simulink subsystem "Gyro_Angles"  (R2023b)
settings: Solver=VariableStepAuto  StartTime=0.0  StopTime=10.0  RelTol=1e-3
undefined symbols (not defined in the file): Gyro_Calibration_Reset_Degree, Gyro_Calibration_Reset_Flag
libraries: simulink_extras x1, simulink x1
settings Model: Creator=ander  LastModifiedBy=ander

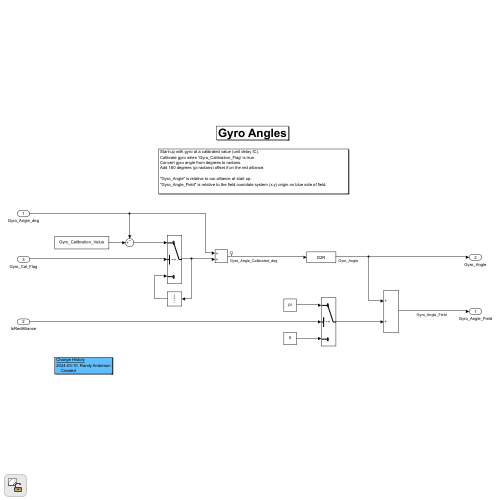
[thumbnail: Simulink's stored preview of the top-level diagram]
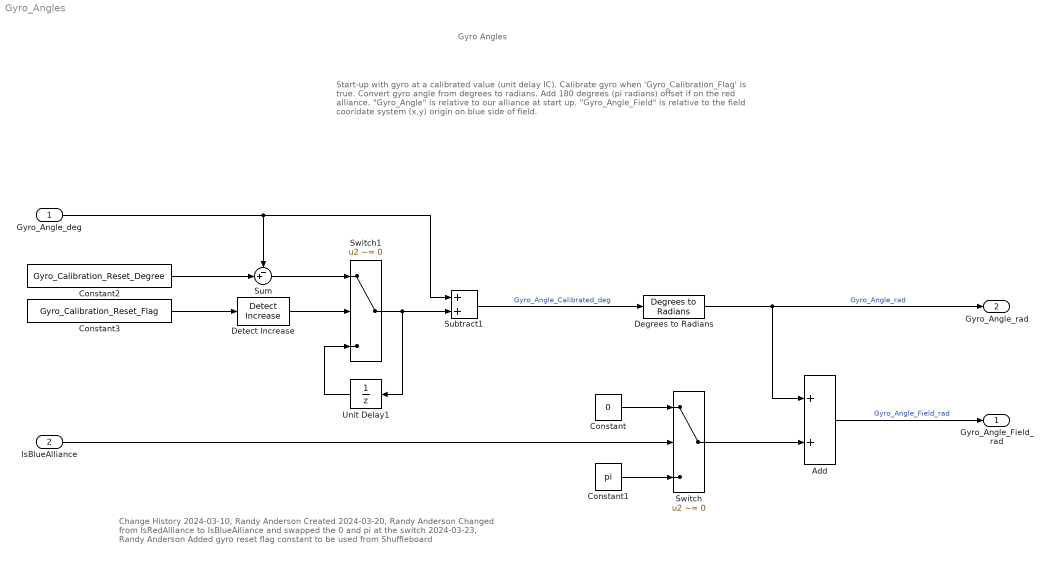
== system Gyro_Angles ==
  note: Gyro Angles
  note: Start-up with gyro at a calibrated value (unit delay IC).
      | Calibrate gyro when 'Gyro_Calibration_Flag' is true.
      | Convert gyro angle from degrees to radians.
      | Add 180 degrees (pi radians) offset if on the red alliance.
      |
      | "Gyro_Angle" is relative to our alliance at start up.
      | "Gyro_Angle_Field" is relative to the field cooridate system (x,y) origin on blue side of field.
  note: Change History
      | 2024-03-10, Randy Anderson
      | Created
      | 2024-03-20, Randy Anderson
      | Changed from IsRedAlliance to IsBlueAlliance and swapped the 0 and pi at the switch
      | 2024-03-23, Randy Anderson
      | Added gyro reset flag constant to be used from Shuffleboard
  Gyro_Angle_deg : Inport
  IsBlueAlliance : Inport  Port=2
  Add : Sum
  Constant : Constant  Value=0
  Constant1 : Constant  Value=pi
  Constant2 : Constant  Value=Gyro_Calibration_Reset_Degree
  Constant3 : Constant  Value=Gyro_Calibration_Reset_Flag
  Degrees to Radians : simulink_extras/Transformations/Degrees to Radians
  Detect Increase : simulink/Logic and Bit Operations/Detect Increase  vinit=0.0  OutDataTypeStr=boolean
  Subtract1 : Sum
  Sum : Sum  Inputs=-+|
  Switch : Switch  Criteria=u2 ~= 0  SaturateOnIntegerOverflow=off  InputSameDT=off
  Switch1 : Switch  Criteria=u2 ~= 0  SaturateOnIntegerOverflow=off  InputSameDT=off
  Unit Delay1 : UnitDelay  InitialCondition=Gyro_Calibration_Reset_Degree  SampleTime=-1  HasFrameUpgradeWarning=on
  Gyro_Angle_Field_rad : Outport
  Gyro_Angle_rad : Outport  Port=2
  wires:
  Add/1 -> Gyro_Angle_Field_rad/1  "Gyro_Angle_Field_rad"
  Degrees to Radians/1 -> Gyro_Angle_rad/1, Add/1  "Gyro_Angle_rad"
  IsBlueAlliance/1 -> Switch/2
  Constant/1 -> Switch/1
  Constant1/1 -> Switch/3
  Unit Delay1/1 -> Switch1/3
  Switch1/1 -> Subtract1/2, Unit Delay1/1
  Sum/1 -> Switch1/1
  Subtract1/1 -> Degrees to Radians/1  "Gyro_Angle_Calibrated_deg"
  Gyro_Angle_deg/1 -> Sum/1, Subtract1/1
  Constant2/1 -> Sum/2
  Switch/1 -> Add/2
  Constant3/1 -> Detect Increase/1
  Detect Increase/1 -> Switch1/2
